simulink model "interleaving_precircuit"  (R2016a)
settings: Solver=ode4  StartTime=0.0  StopTime=Tfinal  FixedStep=Ts  RelTol=1e-3
values from neighbouring files (symbols this model uses):
  delta = acos(Ef/Vt)    [sim_parameters.m]    (also in sim_parameters_parallel.m; sim_parameters_rl_load.m = 0)
  fsw = 10e3    (= 10000)    [sim_parameters.m]    (also in sim_parameters_parallel.m; sim_parameters_rl_load.m)
  Ts = 1e-6    (= 1e-06)    [sim_parameters.m]    (also in sim_parameters_parallel.m = 1e-07; sim_parameters_rl_load.m = 1e-08)
  wout = 2*pi*fout    (= 314.159265359)    [sim_parameters.m]    (also in sim_parameters_parallel.m; sim_parameters_rl_load.m)
undefined symbols (not defined in the file or in its folder): Cdcrec, ma1
libraries: powerlib x23, powerlib_meascontrol x16
settings Model: SimulationMode=accelerator  Creator=ugurm  LastModifiedBy=mesutto
settings DataIOCC: LimitDataPoints=on  SaveFormat=Array
settings DebuggingCC: UnderspecifiedInitializationDetection=Classic  MergeDetectMultiDrivingBlocksExec=none  SolverPrmCheckMsg=warning  StateNameClashWarn=warning
settings HardwareCC: ProdBitPerPointer=32  ProdLargestAtomicFloat=None  ProdIntDivRoundTo=Undefined  ProdEndianess=Unspecified  ProdWordSize=32  ProdHWDeviceType=32-bit Generic
settings ModelReferenceCC: PropagateSignalLabelsOutOfModel=off
settings ConfigComp: CovModelRefEnable=Off

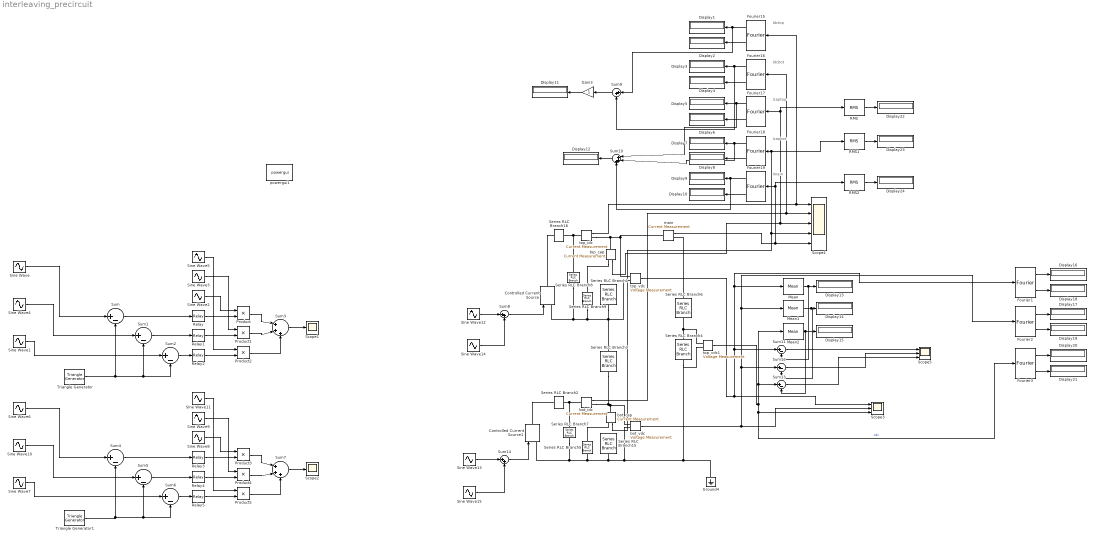
== system interleaving_precircuit ==
  note: Idctop
  note: Idcbot
  note: Icaptop
  note: Icapbot
  note: Imain
  Controlled Current Source : powerlib/Electrical Sources/Controlled Current Source  Initialize=off  Source_Type=AC  Amplitude=0  Phase=0  Frequency=0  Measurements=None
  Controlled Current Source1 : powerlib/Electrical Sources/Controlled Current Source  Initialize=off  Source_Type=AC  Amplitude=0  Phase=0  Frequency=0  Measurements=None
  Display{1..24} (24 alike) : Display
  Fourier{1..3,15..19} (8 alike) : powerlib_meascontrol/Measurements/Fourier  Freq=fsw  n=1  InInit=[0, 0]  Ts=0
  Gain3 : Gain
  Ground4 : powerlib/Elements/Ground  LConnTagsString=a
  Mean : powerlib_meascontrol/Measurements/Mean  Freq=fsw  Vinit=0  Ts=0
  Mean1 : powerlib_meascontrol/Measurements/Mean  Freq=fsw  Vinit=0  Ts=0
  Mean2 : powerlib_meascontrol/Measurements/Mean  Freq=fsw  Vinit=0  Ts=0
  Product{,1..5} (6 alike) : Product
  RMS : powerlib_meascontrol/Measurements/RMS  TrueRMS=on  Freq=fsw  RMSInit=0  Ts=0
  RMS1 : powerlib_meascontrol/Measurements/RMS  TrueRMS=on  Freq=fsw  RMSInit=0  Ts=0
  RMS2 : powerlib_meascontrol/Measurements/RMS  TrueRMS=on  Freq=fsw  RMSInit=0  Ts=0
  Relay{,1..5} (6 alike) : Relay
  Scope1 : Scope
  Scope2 : Scope
  Scope3 : Scope  NumInputPorts=3
  Scope4 : Scope  NumInputPorts=5
  Scope5 : Scope  NumInputPorts=3
  Series RLC Branch1 : powerlib/Elements/Series RLC Branch  LConnTagsString=__new0  RConnTagsString=__new0  BranchType=RLC  Resistance=20e-3  Inductance=20e-9  SetiL0=off  InitialCurrent=0  Capacitance=15e-6  Setx0=off  InitialVoltage=270  Measurements=None
  Series RLC Branch15 : powerlib/Elements/Series RLC Branch  LConnTagsString=__new0  RConnTagsString=__new0  BranchType=RLC  Resistance=20e-3  Inductance=20e-9  SetiL0=off  InitialCurrent=0  Capacitance=15e-6  Setx0=off  InitialVoltage=270  Measurements=None
  Series RLC Branch16 : powerlib/Elements/Series RLC Branch  LConnTagsString=__new0  RConnTagsString=__new0  BranchType=R  Resistance=1e-6  Inductance=1e-12  SetiL0=off  InitialCurrent=0  Capacitance=Cdcrec  Setx0=on  InitialVoltage=270  Measurements=None
  Series RLC Branch2 : powerlib/Elements/Series RLC Branch  LConnTagsString=__new0  RConnTagsString=__new0  BranchType=R  Resistance=1e-6  Inductance=1e-12  SetiL0=off  InitialCurrent=0  Capacitance=Cdcrec  Setx0=on  InitialVoltage=270  Measurements=None
  Series RLC Branch3 : powerlib/Elements/Series RLC Branch  LConnTagsString=__new0  RConnTagsString=__new0  BranchType=RL  Resistance=0.1  Inductance=1e-6  SetiL0=off  InitialCurrent=0  Capacitance=Cdcrec  Setx0=on  InitialVoltage=270  Measurements=None
  Series RLC Branch4 : powerlib/Elements/Series RLC Branch  LConnTagsString=__new0  RConnTagsString=__new0  BranchType=RLC  Resistance=200e-3  Inductance=200e-9  SetiL0=off  InitialCurrent=0  Capacitance=2e-3  Setx0=off  InitialVoltage=270  Measurements=None
  Series RLC Branch5 : powerlib/Elements/Series RLC Branch  LConnTagsString=__new0  RConnTagsString=__new0  BranchType=C  Resistance=20e-3  Inductance=20e-9  SetiL0=off  InitialCurrent=0  Capacitance=15e-6  Setx0=off  InitialVoltage=270  Measurements=None
  Series RLC Branch6 : powerlib/Elements/Series RLC Branch  LConnTagsString=__new0  RConnTagsString=__new0  BranchType=RL  Resistance=0.1  Inductance=1e-6  SetiL0=off  InitialCurrent=0  Capacitance=Cdcrec  Setx0=on  InitialVoltage=270  Measurements=None
  Series RLC Branch7 : powerlib/Elements/Series RLC Branch  LConnTagsString=__new0  RConnTagsString=__new0  BranchType=R  Resistance=1e9  Inductance=1e-12  SetiL0=off  InitialCurrent=0  Capacitance=Cdcrec  Setx0=on  InitialVoltage=270  Measurements=None
  Series RLC Branch8 : powerlib/Elements/Series RLC Branch  LConnTagsString=__new0  RConnTagsString=__new0  BranchType=R  Resistance=1e9  Inductance=1e-12  SetiL0=off  InitialCurrent=0  Capacitance=Cdcrec  Setx0=on  InitialVoltage=270  Measurements=None
  Series RLC Branch9 : powerlib/Elements/Series RLC Branch  LConnTagsString=__new0  RConnTagsString=__new0  BranchType=C  Resistance=20e-3  Inductance=20e-9  SetiL0=off  InitialCurrent=0  Capacitance=15e-6  Setx0=off  InitialVoltage=270  Measurements=None
  Sine Wave : Sin  Amplitude=ma1  Frequency=wout  Phase=delta  SampleTime=0
  Sine Wave1 : Sin  Amplitude=ma1  Frequency=wout  Phase=2*pi/3+delta  SampleTime=0
  Sine Wave10 : Sin  Amplitude=ma1  Frequency=wout  Phase=-2*pi/3+delta  SampleTime=0
  Sine Wave11 : Sin  Amplitude=10  Frequency=wout  Phase=2*pi/3  SampleTime=0
  Sine Wave12 : Sin  Amplitude=5  Frequency=2*pi*fsw  SampleTime=0
  Sine Wave13 : Sin  Amplitude=5  Frequency=2*pi*fsw  Phase=pi  SampleTime=0
  Sine Wave14 : Sin  Amplitude=5  Frequency=2*pi*fsw*2  SampleTime=0
  Sine Wave15 : Sin  Amplitude=5  Frequency=2*pi*fsw*2  SampleTime=0
  Sine Wave2 : Sin  Amplitude=10  Frequency=wout  SampleTime=0
  Sine Wave3 : Sin  Amplitude=10  Frequency=wout  Phase=-2*pi/3  SampleTime=0
  Sine Wave4 : Sin  Amplitude=ma1  Frequency=wout  Phase=-2*pi/3+delta  SampleTime=0
  Sine Wave5 : Sin  Amplitude=10  Frequency=wout  Phase=2*pi/3  SampleTime=0
  Sine Wave6 : Sin  Amplitude=ma1  Frequency=wout  Phase=delta  SampleTime=0
  Sine Wave7 : Sin  Amplitude=ma1  Frequency=wout  Phase=2*pi/3+delta  SampleTime=0
  Sine Wave8 : Sin  Amplitude=10  Frequency=wout  SampleTime=0
  Sine Wave9 : Sin  Amplitude=10  Frequency=wout  Phase=-2*pi/3  SampleTime=0
  Sum{,1..2,4..6,11..13} (9 alike) : Sum  Inputs=|+-
  Sum10 : Sum  Inputs=|+++
  Sum14 : Sum  Inputs=|++
  Sum3 : Sum  Inputs=|+++
  Sum7 : Sum  Inputs=|+++
  Sum8 : Sum  Inputs=|++
  Sum9 : Sum  Inputs=|++
  Triangle Generator : powerlib_meascontrol/Pulse & Signal Generators/Triangle Generator  Freq=fsw  Phase=0  Ts=Ts
  Triangle Generator1 : powerlib_meascontrol/Pulse & Signal Generators/Triangle Generator  Freq=fsw  Phase=0  Ts=Ts
  bot_cap : powerlib/Measurements/Current Measurement  PhasorSimulation=off  OutputType=Complex  PSBequivalent=0
  bot_idc : powerlib/Measurements/Current Measurement  PhasorSimulation=off  OutputType=Complex  PSBequivalent=0
  bot_vdc : powerlib/Measurements/Voltage Measurement  PhasorSimulation=off  OutputType=Complex  PSBequivalent=0
  main : powerlib/Measurements/Current Measurement  PhasorSimulation=off  OutputType=Complex  PSBequivalent=0
  powergui1 : powerlib/powergui  Priority=1  SimulationMode=Discrete  SolverType=Tustin  SampleTime=Ts  frequency=60  SPID=off  DisableSnubberDevices=off  DisableRonSwitches=off  DisableVfSwitches=off  SwTol=0  DisplayEquations=off  Interpol=off  ExternalGateDelay=off  methode=off  Ts=0  FunctionMessages=off  echomessages=off  HookPort=off  EnableUseOfTLC=off  x0status=blocks  frequencyindice=0  Pbase=100e6  ErrMax=1e-4  Iterations=50  UnitsV=kV  UnitsW=MW  buscounter=0  RestoreLinks=warning  ResistiveCurrentMeasurement=off  Frange=[0:2:500]  Ylog=off  Xlog=on  ShowGrid=off  save=off  variable=ZData  structure=newidcs  ZoomFFT=off  StartTime=0.04  cycles=5  DisplayStyle=6  fundamental=50  FreqAxis=off  MaxFrequency=600  frequencyindicesteady=1  RmsSteady=1  display=off
  top_cap : powerlib/Measurements/Current Measurement  PhasorSimulation=off  OutputType=Complex  PSBequivalent=0
  top_idc : powerlib/Measurements/Current Measurement  PhasorSimulation=off  OutputType=Complex  PSBequivalent=0
  top_vdc : powerlib/Measurements/Voltage Measurement  PhasorSimulation=off  OutputType=Complex  PSBequivalent=0
  top_vdc1 : powerlib/Measurements/Voltage Measurement  PhasorSimulation=off  OutputType=Complex  PSBequivalent=0
  wires:
  Triangle Generator/1 -> Sum1/2, Sum2/2, Sum/2
  Sine Wave4/1 -> Sum1/1
  Sine Wave1/1 -> Sum2/1
  Sum/1 -> Relay/1
  Sum1/1 -> Relay1/1
  Sum2/1 -> Relay2/1
  Sine Wave/1 -> Sum/1
  Relay/1 -> Product/2
  Relay2/1 -> Product2/2
  Sine Wave2/1 -> Product/1
  Relay1/1 -> Product1/2
  Sine Wave3/1 -> Product1/1
  Sine Wave5/1 -> Product2/1
  Product1/1 -> Sum3/2
  Product/1 -> Sum3/1
  Product2/1 -> Sum3/3
  Sum3/1 -> Scope1/1
  Triangle Generator1/1 -> Sum5/2, Sum6/2, Sum4/2
  Sine Wave10/1 -> Sum5/1
  Sine Wave7/1 -> Sum6/1
  Sum4/1 -> Relay3/1
  Sum5/1 -> Relay4/1
  Sum6/1 -> Relay5/1
  Sine Wave6/1 -> Sum4/1
  Relay3/1 -> Product3/2
  Relay5/1 -> Product5/2
  Sine Wave8/1 -> Product3/1
  Relay4/1 -> Product4/2
  Sine Wave9/1 -> Product4/1
  Sine Wave11/1 -> Product5/1
  Product4/1 -> Sum7/2
  Product3/1 -> Sum7/1
  Product5/1 -> Sum7/3
  Sum7/1 -> Scope2/1
  top_vdc1/1 -> Fourier3/1, Scope3/3, Mean2/1, Sum13/1  "vdc"
  bot_idc/1 -> Fourier16/1, Scope4/2
  top_cap/1 -> Scope4/3, RMS/1, Fourier17/1
  main/1 -> RMS2/1, Fourier19/1, Scope4/5
  Fourier15/1 -> Sum9/1, Display1/1
  Fourier15/2 -> Display2/1
  top_idc/1 -> Fourier15/1, Scope4/1
  Fourier16/1 -> Sum9/2, Display3/1
  Fourier16/2 -> Display4/1
  Fourier17/2 -> Display6/1
  Fourier18/1 -> Sum10/2, Display7/1
  Fourier18/2 -> Display8/1
  bot_cap/1 -> RMS1/1, Fourier18/1, Scope4/4
  Fourier19/1 -> Sum10/3, Display9/1
  Fourier19/2 -> Display10/1
  Sum9/1 -> Gain3/1
  Sum10/1 -> Display12/1
  Fourier17/1 -> Sum10/1, Display5/1
  Gain3/1 -> Display11/1
  Mean/1 -> Sum11/2, Display13/1
  Mean1/1 -> Sum12/2, Display14/1
  Mean2/1 -> Sum13/2, Display15/1
  Sum11/1 -> Scope5/1
  bot_vdc/1 -> Scope3/2, Sum12/1, Fourier2/1, Mean1/1
  Sum12/1 -> Scope5/2
  Sum13/1 -> Scope5/3
  Fourier1/1 -> Display16/1
  Fourier1/2 -> Display18/1
  Fourier2/1 -> Display17/1
  Fourier2/2 -> Display19/1
  Fourier3/1 -> Display20/1
  Fourier3/2 -> Display21/1
  top_vdc/1 -> Sum11/1, Fourier1/1, Mean/1, Scope3/1
  Sine Wave12/1 -> Sum8/1
  Sine Wave14/1 -> Sum8/2
  Sine Wave13/1 -> Sum14/1
  Sine Wave15/1 -> Sum14/2
  Sum8/1 -> Controlled Current Source/1
  Sum14/1 -> Controlled Current Source1/1
  RMS/1 -> Display22/1
  RMS1/1 -> Display23/1
  RMS2/1 -> Display24/1
  connections:
  top_cap/LConn1 -- top_vdc/LConn2 -- main/LConn1 -- top_idc/RConn1
  Series RLC Branch1/RConn1 -- top_vdc/LConn1 -- Series RLC Branch3/LConn1 -- Series RLC Branch9/RConn1 -- Controlled Current Source/LConn1 -- Series RLC Branch8/LConn1
  Series RLC Branch3/RConn1 -- bot_idc/RConn1 -- bot_cap/LConn1 -- bot_vdc/LConn2
  bot_vdc/LConn1 -- top_vdc1/LConn1 -- Series RLC Branch4/RConn1 -- Ground4/LConn1 -- Series RLC Branch15/RConn1 -- Series RLC Branch5/RConn1 -- Series RLC Branch7/LConn1 -- Controlled Current Source1/LConn1
  Series RLC Branch6/LConn1 -- main/RConn1
  Series RLC Branch4/LConn1 -- top_vdc1/LConn2 -- Series RLC Branch6/RConn1
  Series RLC Branch2/RConn1 -- Controlled Current Source1/RConn1
  top_idc/LConn1 -- Series RLC Branch8/RConn1 -- Series RLC Branch16/LConn1
  bot_idc/LConn1 -- Series RLC Branch7/RConn1 -- Series RLC Branch2/LConn1
  Series RLC Branch16/RConn1 -- Controlled Current Source/RConn1
  Series RLC Branch5/LConn1 -- bot_cap/RConn1
  top_cap/RConn1 -- Series RLC Branch9/LConn1
